simulink model "PMSM_FOC_INVERTER_COMPARISON"  (R2023b)
settings: Solver=VariableStepAuto  StartTime=0.0  StopTime=1  RelTol=1e-3
InitFcn:
  | Ld = 1.7e-3;
  | Lq = 3.2e-3;
  | Rs = 0.02;
  | Lambda_m = 0.2205;
  | J = 0.0027;
  | P = 4;
  | B = 0.001;
  | Vdc = 500;
libraries: slpidlib x9, spsControlledVoltageSourceLib x3, spsGroundLib x3, spsVoltageMeasurementLib x3, spsDCVoltageSourceLib x1, spsPermanentMagnetSynchronousMachineLib x1, spsUniversalBridgeLib x1, sps_lib x1, spsTriangleGeneratorLib x1
(part 1 of 2)
settings Model: Creator=Nabil  LastModifiedBy=Nabil

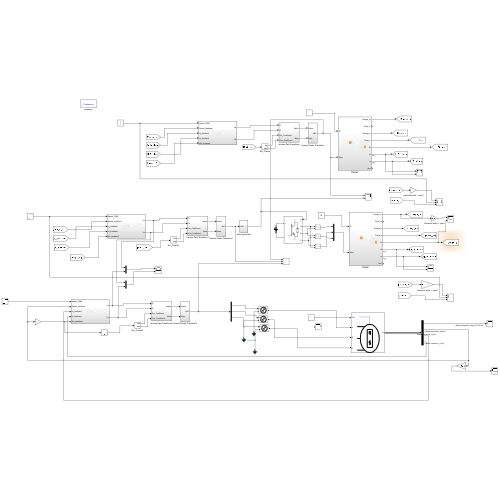
[thumbnail: Simulink's stored preview of the top-level diagram]
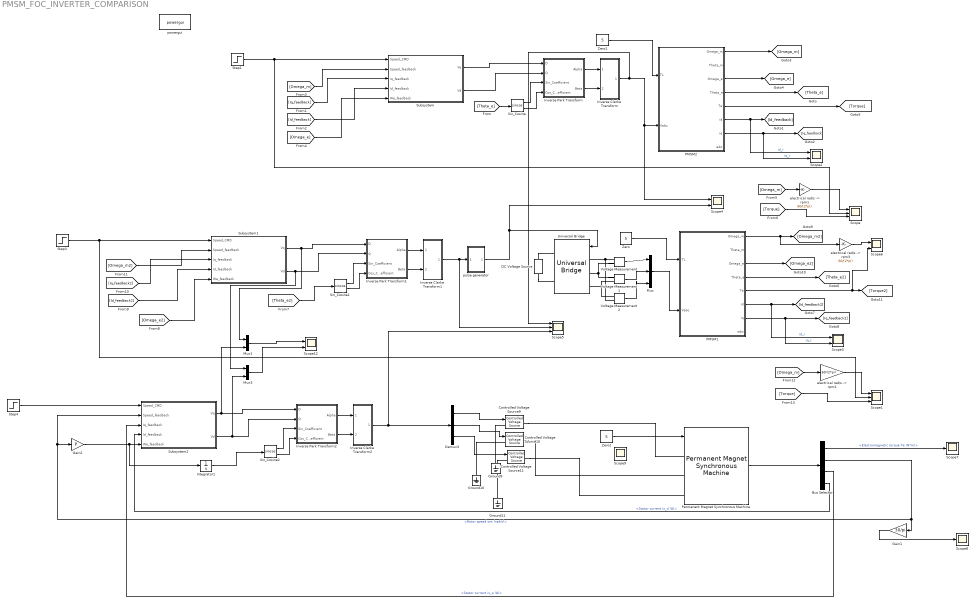
== system PMSM_FOC_INVERTER_COMPARISON ==
  Bus Selector : BusSelector  OutputSignals=Electromagnetic torque Te (N*m),Rotor speed wm (rad/s),Stator current is_q (A),Stator current is_d (A)
  Controlled Voltage Source10 : spsControlledVoltageSourceLib/Controlled Voltage Source  Initialize=on  Source_Type=AC  Amplitude=0  Phase=0  Frequency=0  Measurements=None
  Controlled Voltage Source11 : spsControlledVoltageSourceLib/Controlled Voltage Source  Initialize=on  Source_Type=AC  Amplitude=0  Phase=0  Frequency=0  Measurements=None
  Controlled Voltage Source9 : spsControlledVoltageSourceLib/Controlled Voltage Source  Initialize=on  Source_Type=AC  Amplitude=0  Phase=0  Frequency=0  Measurements=None
  DC Voltage Source : spsDCVoltageSourceLib/DC Voltage Source  Amplitude=Vdc  Measurements=None
  Demux3 : Demux  Outputs=3
  Gain1 : Gain  Gain=30/pi
  Gain2 : Gain  Gain=P
  Ground10 : spsGroundLib/Ground  LConnTagsString=a
  Ground11 : spsGroundLib/Ground  LConnTagsString=a
  Ground9 : spsGroundLib/Ground  LConnTagsString=a
  Integrator1 : Integrator
  Inverse Clarke Transform : Subsystem
  Inverse Clarke Transform1 : Subsystem
  Inverse Clarke Transform2 : Subsystem
  Inverse Park Transform : Subsystem
  Inverse Park Transform1 : Subsystem
  Inverse Park Transform2 : Subsystem
  Mux : Mux  Inputs=3
  Mux1 : Mux  Inputs=2
  Mux3 : Mux  Inputs=2
  PMSM1 : Subsystem
  PMSM2 : Subsystem
  Permanent Magnet Synchronous Machine : spsPermanentMagnetSynchronousMachineLib/Permanent Magnet Synchronous Machine  NbPhases=3  FluxDistribution=Sinusoidal  RotorType=Round  MechanicalLoad=Torque Tm  PresetModel=No  ShowDetailedParameters=on  MeasurementBus=off  Resistance=0.0485  Inductance=8.5e-3  dqInductances=[8.5e-3,8.5e-3]  La=0.000395  MachineConstant=Flux linkage established by magnets (V.s)  Flux=0.1194  VoltageCst=86.6271  TorqueCst=0.7164  Flat=120  Mechanical=[0.0027 0.0004924 4 0]  PolePairs=4  InitialConditions=[0,0, 0,0]  InitialConditions5ph=[0 0 0 0 0 0]  RefAngle=90 degrees behind phase A axis (modified Park)  IterativeDiscreteModel=Trapezoidal non iterative  TsBlock=-1  TsPowergui=0
  Scope : Scope  NumInputPorts=3
  Scope1 : Scope  NumInputPorts=3
  Scope{2..4,6,12} (5 alike) : Scope  NumInputPorts=2
  Scope5 : Scope  NumInputPorts=3
  Scope7 : Scope
  Scope8 : Scope
  Scope9 : Scope
  Sin_Cosine : Trigonometry  Operator=sincos
  Sin_Cosine1 : Trigonometry  Operator=sincos
  Sin_Cosine2 : Trigonometry  Operator=sincos
  Step1 : Step  Time=0.7  Before=500  After=1000  SampleTime=0
  Step3 : Step  Time=0.7  Before=500  After=1000  SampleTime=0
  Step4 : Step  Time=0.7  Before=500  After=1000  SampleTime=0
  Subsystem : Subsystem
  Subsystem1 : Subsystem
  Subsystem2 : Subsystem
  Universal Bridge : spsUniversalBridgeLib/Universal Bridge  Arms=3  SnubberResistance=1e5  SnubberCapacitance=inf  Device=IGBT / Diodes  Ron=1e-3  Lon=0  ForwardVoltages="[  0  0  ]"  ForwardVoltage=0  GTOparameters=[ 10e-6 , 20e-6 ]  IGBTparameters=[ 1e-6 , 2e-6 ]  Measurements=None  Measurements_2=None  converterType=Rectifier
  Voltage Measurement : spsVoltageMeasurementLib/Voltage Measurement  PhasorSimulation=off  OutputType=Complex  PSBequivalent=0
  Voltage Measurement1 : spsVoltageMeasurementLib/Voltage Measurement  PhasorSimulation=off  OutputType=Complex  PSBequivalent=0
  Voltage Measurement2 : spsVoltageMeasurementLib/Voltage Measurement  PhasorSimulation=off  OutputType=Complex  PSBequivalent=0
  Zero : Constant  Value=5  OutDataTypeStr=Inherit: Inherit via back propagation
  Zero1 : Constant  Value=5  OutDataTypeStr=Inherit: Inherit via back propagation
  Zero2 : Constant  Value=5  OutDataTypeStr=Inherit: Inherit via back propagation
  "electrical rad/s -> rpm1" : Gain  Gain=60/(2*pi)
  "electrical rad/s -> rpm2" : Gain  Gain=60/(2*pi)
  "electrical rad/s -> rpm3" : Gain  Gain=60/(2*pi)
  powergui : sps_lib/powergui  Priority=1  SimulationMode=Continuous  SampleTime=50e-6  frequency=60  Iterations=50  frequencyindice=0  Pbase=100e6  ErrMax=1e-4  UnitsV=kV  UnitsW=MW  buscounter=0  FunctionMessages=off  echomessages=off  EnableUseOfTLC=off  CurrentSourceSwitches=off  DisableSnubberDevices=off  DisableRonSwitches=off  DisableVfSwitches=off  DisplayEquations=off  AutomaticDiscreteSolvers=off  SolverType=Tustin/Backward Euler (TBE)  Interpol=off  ExternalGateDelay=off  methode=off  Ts=100  x0status=blocks  SPID=on  SwTol=0  HookPort=off  NonlinearTolerance=1e-4  nMaxIteration=100  ContinueOnMaxIteration=off  RestoreLinks=warning  ResistiveCurrentMeasurement=off  Frange=[0:2:500]  Ylog=off  Xlog=on  ShowGrid=off  save=off  variable=ZData  structure=0  ZoomFFT=off  StartTime=0.0  cycles=1  DisplayStyle=1  fundamental=60  FreqAxis=off  MaxFrequency=1000  frequencyindicesteady=1  RmsSteady=1  display=off
  pulse generator : Subsystem
  wires:
  [Theta_e] -> Sin_Cosine/1
  Sin_Cosine/2 -> Inverse Park Transform/4(Cos_Coefficient)
  Sin_Cosine/1 -> Inverse Park Transform/3(Sin_Coefficient)
  Inverse Park Transform/2(Beta) -> Inverse Clarke Transform/2(Beta)
  Inverse Park Transform/1(Alpha) -> Inverse Clarke Transform/1(Alpha)
  PMSM2/4(Theta_e) -> [Theta_e]
  Subsystem/1(Vq) -> Inverse Park Transform/1(D)
  Subsystem/2(Vd) -> Inverse Park Transform/2(Q)
  Step1/1 -> Scope/2, Subsystem/1(Speed_CMD)
  PMSM2/7(iq) -> Scope2/2, [Iq_feedback]  "iq_r"
  PMSM2/6(id) -> Scope2/1, [Id_feedback]  "id_r"
  [Iq_feedback] -> Subsystem/3(Iq_feedback)
  [Id_feedback] -> Subsystem/4(Id_feedback)
  PMSM2/1(Omega_m) -> [Omega_m]
  [Omega_m] -> Subsystem/2(Speed_feedback)
  PMSM2/3(Omega_e) -> [Omega_e]
  [Omega_e] -> Subsystem/5(We_feedback)
  PMSM2/5(Te) -> [Torque]
  [Torque] -> Scope/3
  Inverse Clarke Transform/1(ABC) -> Scope5/1, Scope4/1, PMSM2/2(Vabc)
  [Omega_m] -> "electrical rad/s -> rpm1"/1
  "electrical rad/s -> rpm1"/1 -> Scope/1
  "electrical rad/s -> rpm2"/1 -> Scope1/1
  [Omega_m] -> "electrical rad/s -> rpm2"/1
  [Torque] -> Scope1/3
  PMSM1/5(Te) -> Scope6/2, [Torque2]
  [Omega_e2] -> Subsystem1/5(We_feedback)
  PMSM1/3(Omega_e) -> [Omega_e2]
  [Omega_m2] -> Subsystem1/2(Speed_feedback)
  PMSM1/1(Omega_m) -> "electrical rad/s -> rpm3"/1, [Omega_m2]
  [Id_feedback2] -> Subsystem1/4(Id_feedback)
  [Iq_feedback2] -> Subsystem1/3(Iq_feedback)
  PMSM1/6(id) -> [Id_feedback2], Scope3/1  "id_r"
  PMSM1/7(iq) -> [Iq_feedback2], Scope3/2  "iq_r"
  Step3/1 -> Scope1/2, Subsystem1/1(Speed_CMD)
  Subsystem1/2(Vd) -> Mux3/1, Inverse Park Transform1/2(Q)
  Subsystem1/1(Vq) -> Mux1/1, Inverse Park Transform1/1(D)
  PMSM1/4(Theta_e) -> [Theta_e2]
  Inverse Park Transform1/1(Alpha) -> Inverse Clarke Transform1/1(Alpha)
  Inverse Park Transform1/2(Beta) -> Inverse Clarke Transform1/2(Beta)
  Sin_Cosine1/1 -> Inverse Park Transform1/3(Sin_Coefficient)
  Sin_Cosine1/2 -> Inverse Park Transform1/4(Cos_Coefficient)
  [Theta_e2] -> Sin_Cosine1/1
  Voltage Measurement/1 -> Mux/1
  Voltage Measurement1/1 -> Mux/2
  Voltage Measurement2/1 -> Mux/3
  Mux/1 -> PMSM1/2(Vabc)
  Inverse Clarke Transform1/1(ABC) -> Scope5/2, pulse generator/1(ABC)
  pulse generator/1(Out1) -> Universal Bridge/1, Scope4/2
  Zero/1 -> PMSM1/1(TL)
  Zero1/1 -> PMSM2/1(TL)
  "electrical rad/s -> rpm3"/1 -> Scope6/1
  Inverse Clarke Transform2/1(ABC) -> Scope5/3, Demux3/1
  Sin_Cosine2/2 -> Inverse Park Transform2/4(Cos_Coefficient)
  Sin_Cosine2/1 -> Inverse Park Transform2/3(Sin_Coefficient)
  Inverse Park Transform2/2(Beta) -> Inverse Clarke Transform2/2(Beta)
  Inverse Park Transform2/1(Alpha) -> Inverse Clarke Transform2/1(Alpha)
  Subsystem2/1(Vq) -> Mux1/2, Inverse Park Transform2/1(D)
  Subsystem2/2(Vd) -> Mux3/2, Inverse Park Transform2/2(Q)
  Zero2/1 -> Permanent Magnet Synchronous Machine/1
  Permanent Magnet Synchronous Machine/1 -> Bus Selector/1
  Bus Selector/1 -> Scope7/1  "<Electromagnetic torque Te (N*m)>"
  Bus Selector/2 -> Gain1/1, Subsystem2/2(Speed_feedback), Gain2/1  "<Rotor speed wm (rad/s)>"
  Bus Selector/3 -> Subsystem2/3(Iq_feedback)  "<Stator current is_q (A)>"
  Bus Selector/4 -> Subsystem2/4(Id_feedback)  "<Stator current is_d (A)>"
  Gain1/1 -> Scope8/1
  Gain2/1 -> Integrator1/1, Subsystem2/5(We_feedback)
  Integrator1/1 -> Sin_Cosine2/1
  Demux3/1 -> Controlled Voltage Source9/1
  Demux3/2 -> Controlled Voltage Source10/1
  Demux3/3 -> Controlled Voltage Source11/1
  Mux1/1 -> Scope12/1
  Mux3/1 -> Scope12/2
  Step4/1 -> Subsystem2/1(Speed_CMD)
  connections:
  DC Voltage Source/RConn1 -- Universal Bridge/RConn1
  DC Voltage Source/LConn1 -- Universal Bridge/RConn2
  Voltage Measurement/LConn1 -- Universal Bridge/LConn1 -- Voltage Measurement2/LConn2
  Voltage Measurement/LConn2 -- Voltage Measurement1/LConn1 -- Universal Bridge/LConn2
  Voltage Measurement1/LConn2 -- Voltage Measurement2/LConn1 -- Universal Bridge/LConn3
  Ground9/LConn1 -- Controlled Voltage Source9/LConn1
  Ground10/LConn1 -- Controlled Voltage Source10/LConn1
  Ground11/LConn1 -- Controlled Voltage Source11/LConn1
  Controlled Voltage Source9/RConn1 -- Permanent Magnet Synchronous Machine/LConn1
  Controlled Voltage Source10/RConn1 -- Permanent Magnet Synchronous Machine/LConn2
  Controlled Voltage Source11/RConn1 -- Permanent Magnet Synchronous Machine/LConn3

== system PMSM_FOC_INVERTER_COMPARISON/Inverse Clarke Transform ==
  note: Inverse Clarke Transform
  note: Converts direct axis (alpha) component and the quadrature axis (beta) component to balanced three-phase quantities
      | The alpha and beta components are dependent on time and speed.
  Alpha : Inport
  Beta : Inport  Port=2
  Add : Sum  Inputs=-+  OutDataTypeStr=Inherit: Same as first input
  Add1 : Sum  Inputs=--  OutDataTypeStr=Inherit: Same as first input
  Gain : Gain  Gain=1/2
  Gain1 : Gain  Gain=sqrt(3)/2
  Mux : Mux  Inputs=3
  ABC : Outport  VectorParamsAs1DForOutWhenUnconnected=off
  wires:
  Beta/1 -> Gain1/1
  Mux/1 -> ABC/1
  Alpha/1 -> Mux/1, Gain/1
  Add1/1 -> Mux/3
  Gain1/1 -> Add1/2, Add/2
  Gain/1 -> Add1/1, Add/1
  Add/1 -> Mux/2

== system PMSM_FOC_INVERTER_COMPARISON/Inverse Clarke Transform1 ==
  note: Converts direct axis (alpha) component and the quadrature axis (beta) component to balanced three-phase quantities
      | The alpha and beta components are dependent on time and speed.
  note: Inverse Clarke Transform
  Alpha : Inport
  Beta : Inport  Port=2
  Add : Sum  Inputs=-+  OutDataTypeStr=Inherit: Same as first input
  Add1 : Sum  Inputs=--  OutDataTypeStr=Inherit: Same as first input
  Gain : Gain  Gain=1/2
  Gain1 : Gain  Gain=sqrt(3)/2
  Mux : Mux  Inputs=3
  ABC : Outport  VectorParamsAs1DForOutWhenUnconnected=off
  wires:
  Add/1 -> Mux/2
  Gain/1 -> Add/1, Add1/1
  Gain1/1 -> Add/2, Add1/2
  Add1/1 -> Mux/3
  Alpha/1 -> Gain/1, Mux/1
  Mux/1 -> ABC/1
  Beta/1 -> Gain1/1

== system PMSM_FOC_INVERTER_COMPARISON/Inverse Clarke Transform2 ==
  note: Inverse Clarke Transform
  note: Converts direct axis (alpha) component and the quadrature axis (beta) component to balanced three-phase quantities
      | The alpha and beta components are dependent on time and speed.
  Alpha : Inport
  Beta : Inport  Port=2
  Add : Sum  Inputs=-+  OutDataTypeStr=Inherit: Same as first input
  Add1 : Sum  Inputs=--  OutDataTypeStr=Inherit: Same as first input
  Gain : Gain  Gain=1/2
  Gain1 : Gain  Gain=sqrt(3)/2
  Mux : Mux  Inputs=3
  ABC : Outport  VectorParamsAs1DForOutWhenUnconnected=off
  wires:
  Beta/1 -> Gain1/1
  Mux/1 -> ABC/1
  Alpha/1 -> Mux/1, Gain/1
  Add1/1 -> Mux/3
  Gain1/1 -> Add1/2, Add/2
  Gain/1 -> Add1/1, Add/1
  Add/1 -> Mux/2

== system PMSM_FOC_INVERTER_COMPARISON/Inverse Park Transform ==
  note: Converts orthogonal rotating reference frame (dq) to two-phase orthogonal stationary reference frame (alpha, beta)
  note: Inverse Park Transform
  D : Inport
  Q : Inport  Port=2
  Sin_Coefficient : Inport  Port=3
  Cos_Coefficient : Inport  Port=4
  Add1 : Sum  Inputs=+-  OutDataTypeStr=Inherit: Same as first input
  Add2 : Sum  OutDataTypeStr=Inherit: Same as first input
  Cos_Coefficient_1 : InportShadow  Port=4
  Product{1..4} (4 alike) : Product  RndMeth=Simplest
  Sin_Coefficient_1 : InportShadow  Port=3
  Alpha : Outport  VectorParamsAs1DForOutWhenUnconnected=off
  Beta : Outport  Port=2  VectorParamsAs1DForOutWhenUnconnected=off
  wires:
  Sin_Coefficient_1/1 -> Product3/2
  Product2/1 -> Add1/2
  Cos_Coefficient_1/1 -> Product4/2
  Add2/1 -> Beta/1
  Product3/1 -> Add2/1
  Add1/1 -> Alpha/1
  Product1/1 -> Add1/1
  Product4/1 -> Add2/2
  Sin_Coefficient/1 -> Product2/2
  D/1 -> Product3/1, Product1/1
  Q/1 -> Product2/1, Product4/1
  Cos_Coefficient/1 -> Product1/2

== system PMSM_FOC_INVERTER_COMPARISON/Inverse Park Transform1 ==
  note: Inverse Park Transform
  note: Converts orthogonal rotating reference frame (dq) to two-phase orthogonal stationary reference frame (alpha, beta)
  D : Inport
  Q : Inport  Port=2
  Sin_Coefficient : Inport  Port=3
  Cos_Coefficient : Inport  Port=4
  Add1 : Sum  Inputs=+-  OutDataTypeStr=Inherit: Same as first input
  Add2 : Sum  OutDataTypeStr=Inherit: Same as first input
  Cos_Coefficient_1 : InportShadow  Port=4
  Product{1..4} (4 alike) : Product  RndMeth=Simplest
  Sin_Coefficient_1 : InportShadow  Port=3
  Alpha : Outport  VectorParamsAs1DForOutWhenUnconnected=off
  Beta : Outport  Port=2  VectorParamsAs1DForOutWhenUnconnected=off
  wires:
  Cos_Coefficient/1 -> Product1/2
  Q/1 -> Product4/1, Product2/1
  D/1 -> Product1/1, Product3/1
  Sin_Coefficient/1 -> Product2/2
  Product4/1 -> Add2/2
  Product1/1 -> Add1/1
  Add1/1 -> Alpha/1
  Product3/1 -> Add2/1
  Add2/1 -> Beta/1
  Cos_Coefficient_1/1 -> Product4/2
  Product2/1 -> Add1/2
  Sin_Coefficient_1/1 -> Product3/2

== system PMSM_FOC_INVERTER_COMPARISON/Inverse Park Transform2 ==
  note: Converts orthogonal rotating reference frame (dq) to two-phase orthogonal stationary reference frame (alpha, beta)
  note: Inverse Park Transform
  D : Inport
  Q : Inport  Port=2
  Sin_Coefficient : Inport  Port=3
  Cos_Coefficient : Inport  Port=4
  Add1 : Sum  Inputs=+-  OutDataTypeStr=Inherit: Same as first input
  Add2 : Sum  OutDataTypeStr=Inherit: Same as first input
  Cos_Coefficient_1 : InportShadow  Port=4
  Product{1..4} (4 alike) : Product  RndMeth=Simplest
  Sin_Coefficient_1 : InportShadow  Port=3
  Alpha : Outport  VectorParamsAs1DForOutWhenUnconnected=off
  Beta : Outport  Port=2  VectorParamsAs1DForOutWhenUnconnected=off
  wires:
  Sin_Coefficient_1/1 -> Product3/2
  Product2/1 -> Add1/2
  Cos_Coefficient_1/1 -> Product4/2
  Add2/1 -> Beta/1
  Product3/1 -> Add2/1
  Add1/1 -> Alpha/1
  Product1/1 -> Add1/1
  Product4/1 -> Add2/2
  Sin_Coefficient/1 -> Product2/2
  D/1 -> Product3/1, Product1/1
  Q/1 -> Product2/1, Product4/1
  Cos_Coefficient/1 -> Product1/2

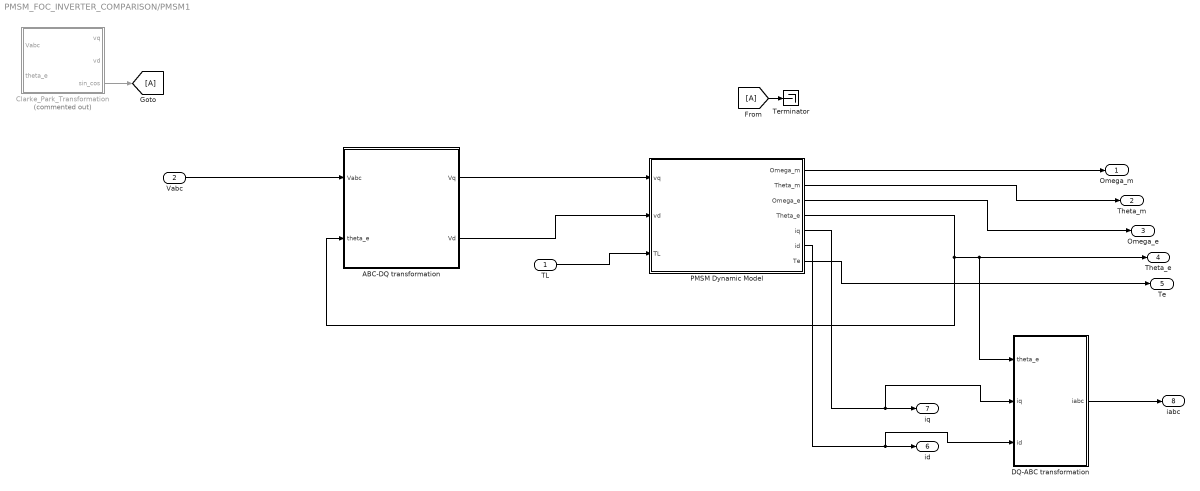
== system PMSM_FOC_INVERTER_COMPARISON/PMSM1 ==
  TL : Inport
  Vabc : Inport  Port=2
  ABC-DQ transformation : Subsystem
  Clarke_Park_Transformation : Subsystem  Commented=on
  DQ-ABC transformation : Subsystem
  From : From
  Goto : Goto
  PMSM Dynamic Model : Subsystem
  Terminator : Terminator
  Omega_m : Outport
  Theta_m : Outport  Port=2
  Omega_e : Outport  Port=3
  Theta_e : Outport  Port=4
  Te : Outport  Port=5
  id : Outport  Port=6
  iq : Outport  Port=7
  iabc : Outport  Port=8
  wires:
  DQ-ABC transformation/1(iabc) -> iabc/1
  ABC-DQ transformation/2(Vd) -> PMSM Dynamic Model/2(vd)
  ABC-DQ transformation/1(Vq) -> PMSM Dynamic Model/1(vq)
  Vabc/1 -> ABC-DQ transformation/1(Vabc)
  PMSM Dynamic Model/3(Omega_e) -> Omega_e/1
  PMSM Dynamic Model/1(Omega_m) -> Omega_m/1
  TL/1 -> PMSM Dynamic Model/3(TL)
  PMSM Dynamic Model/4(Theta_e) -> Theta_e/1, DQ-ABC transformation/1(theta_e), ABC-DQ transformation/2(theta_e)
  Clarke_Park_Transformation/3(sin_cos) -> Goto/1
  PMSM Dynamic Model/5(iq) -> iq/1, DQ-ABC transformation/2(iq)
  PMSM Dynamic Model/6(id) -> id/1, DQ-ABC transformation/3(id)
  PMSM Dynamic Model/7(Te) -> Te/1
  PMSM Dynamic Model/2(Theta_m) -> Theta_m/1
  From/1 -> Terminator/1

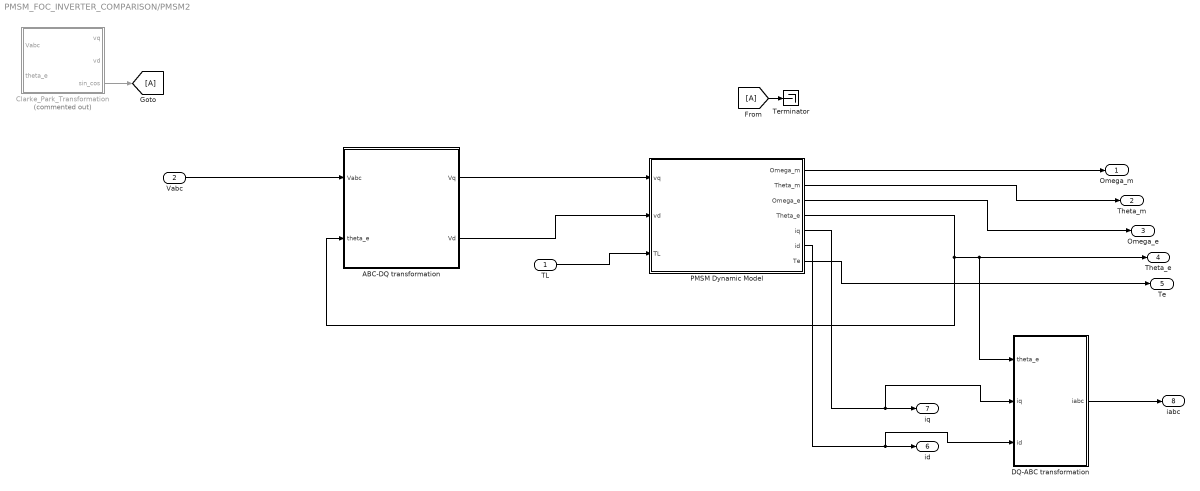
== system PMSM_FOC_INVERTER_COMPARISON/PMSM2 ==
  TL : Inport
  Vabc : Inport  Port=2
  ABC-DQ transformation : Subsystem
  Clarke_Park_Transformation : Subsystem  Commented=on
  DQ-ABC transformation : Subsystem
  From : From
  Goto : Goto
  PMSM Dynamic Model : Subsystem
  Terminator : Terminator
  Omega_m : Outport
  Theta_m : Outport  Port=2
  Omega_e : Outport  Port=3
  Theta_e : Outport  Port=4
  Te : Outport  Port=5
  id : Outport  Port=6
  iq : Outport  Port=7
  iabc : Outport  Port=8
  wires:
  From/1 -> Terminator/1
  PMSM Dynamic Model/2(Theta_m) -> Theta_m/1
  PMSM Dynamic Model/7(Te) -> Te/1
  PMSM Dynamic Model/6(id) -> DQ-ABC transformation/3(id), id/1
  PMSM Dynamic Model/5(iq) -> DQ-ABC transformation/2(iq), iq/1
  Clarke_Park_Transformation/3(sin_cos) -> Goto/1
  PMSM Dynamic Model/4(Theta_e) -> ABC-DQ transformation/2(theta_e), DQ-ABC transformation/1(theta_e), Theta_e/1
  TL/1 -> PMSM Dynamic Model/3(TL)
  PMSM Dynamic Model/1(Omega_m) -> Omega_m/1
  PMSM Dynamic Model/3(Omega_e) -> Omega_e/1
  Vabc/1 -> ABC-DQ transformation/1(Vabc)
  ABC-DQ transformation/1(Vq) -> PMSM Dynamic Model/1(vq)
  ABC-DQ transformation/2(Vd) -> PMSM Dynamic Model/2(vd)
  DQ-ABC transformation/1(iabc) -> iabc/1

== system PMSM_FOC_INVERTER_COMPARISON/Subsystem ==
  Speed_CMD : Inport
  Speed_feedback : Inport  Port=2
  Iq_feedback : Inport  Port=3
  Id_feedback : Inport  Port=4
  We_feedback : Inport  Port=5
  Current Controller : Subsystem
  Subsystem : Subsystem
  "electrical rad/s -> rpm1" : Gain  Gain=60/(2*pi)
  Vq : Outport
  Vd : Outport  Port=2
  wires:
  Speed_CMD/1 -> Subsystem/1(Speed_CMD)
  Subsystem/1(Iq_ref) -> Current Controller/1(iq_reference)
  Subsystem/2(Id_ref) -> Current Controller/2(id_reference)
  We_feedback/1 -> Current Controller/5(spd_we)
  Current Controller/1(vd_reference) -> Vq/1
  Current Controller/2(vq_reference) -> Vd/1
  Iq_feedback/1 -> Current Controller/4(iq_feedback)
  Id_feedback/1 -> Current Controller/3(id_feedback)
  Speed_feedback/1 -> "electrical rad/s -> rpm1"/1
  "electrical rad/s -> rpm1"/1 -> Subsystem/2(Speed_feedback)

== system PMSM_FOC_INVERTER_COMPARISON/Subsystem1 ==
  Speed_CMD : Inport
  Speed_feedback : Inport  Port=2
  Iq_feedback : Inport  Port=3
  Id_feedback : Inport  Port=4
  We_feedback : Inport  Port=5
  Current Controller : Subsystem
  Subsystem : Subsystem
  "electrical rad/s -> rpm1" : Gain  Gain=60/(2*pi)
  Vq : Outport
  Vd : Outport  Port=2
  wires:
  "electrical rad/s -> rpm1"/1 -> Subsystem/2(Speed_feedback)
  Speed_feedback/1 -> "electrical rad/s -> rpm1"/1
  Id_feedback/1 -> Current Controller/3(id_feedback)
  Iq_feedback/1 -> Current Controller/4(iq_feedback)
  Current Controller/2(vq_reference) -> Vd/1
  Current Controller/1(vd_reference) -> Vq/1
  We_feedback/1 -> Current Controller/5(spd_we)
  Subsystem/2(Id_ref) -> Current Controller/2(id_reference)
  Subsystem/1(Iq_ref) -> Current Controller/1(iq_reference)
  Speed_CMD/1 -> Subsystem/1(Speed_CMD)

== system PMSM_FOC_INVERTER_COMPARISON/Subsystem2 ==
  Speed_CMD : Inport
  Speed_feedback : Inport  Port=2
  Iq_feedback : Inport  Port=3
  Id_feedback : Inport  Port=4
  We_feedback : Inport  Port=5
  Current Controller : Subsystem
  Subsystem : Subsystem
  "electrical rad/s -> rpm1" : Gain  Gain=60/(2*pi)
  Vq : Outport
  Vd : Outport  Port=2
  wires:
  Speed_CMD/1 -> Subsystem/1(Speed_CMD)
  Subsystem/1(Iq_ref) -> Current Controller/1(iq_reference)
  Subsystem/2(Id_ref) -> Current Controller/2(id_reference)
  We_feedback/1 -> Current Controller/5(spd_we)
  Current Controller/1(vd_reference) -> Vq/1
  Current Controller/2(vq_reference) -> Vd/1
  Iq_feedback/1 -> Current Controller/4(iq_feedback)
  Id_feedback/1 -> Current Controller/3(id_feedback)
  Speed_feedback/1 -> "electrical rad/s -> rpm1"/1
  "electrical rad/s -> rpm1"/1 -> Subsystem/2(Speed_feedback)

== system PMSM_FOC_INVERTER_COMPARISON/pulse generator ==
  ABC : Inport
  Demux : Demux  Outputs=3
  Gain : Gain  Gain=1/Vdc
  Gain1 : Gain  Gain=1/Vdc
  Gain2 : Gain  Gain=1/Vdc
  Mux : Mux  Inputs=6
  NOT : Logic  Operator=NOT  IconShape=distinctive  AllPortsSameDT=off  OutDataTypeStr=boolean
  NOT1 : Logic  Operator=NOT  IconShape=distinctive  AllPortsSameDT=off  OutDataTypeStr=boolean
  NOT2 : Logic  Operator=NOT  IconShape=distinctive  AllPortsSameDT=off  OutDataTypeStr=boolean
  Relational Operator : RelationalOperator  OutDataTypeStr=boolean  RndMeth=Simplest  InputSameDT=off
  Relational Operator1 : RelationalOperator  OutDataTypeStr=boolean  RndMeth=Simplest  InputSameDT=off
  Relational Operator2 : RelationalOperator  OutDataTypeStr=boolean  RndMeth=Simplest  InputSameDT=off
  Triangle Generator : spsTriangleGeneratorLib/Triangle Generator  Freq=1e4  Phase=0  Ts=0
  Out1 : Outport
  wires:
  Gain/1 -> Relational Operator/1
  Demux/2 -> Gain1/1
  Demux/3 -> Gain2/1
  Gain2/1 -> Relational Operator2/1
  Gain1/1 -> Relational Operator1/1
  Triangle Generator/1 -> Relational Operator/2, Relational Operator1/2, Relational Operator2/2
  Relational Operator/1 -> Mux/1, NOT/1
  NOT/1 -> Mux/2
  Relational Operator1/1 -> Mux/3, NOT1/1
  NOT1/1 -> Mux/4
  Relational Operator2/1 -> Mux/5, NOT2/1
  NOT2/1 -> Mux/6
  Mux/1 -> Out1/1
  ABC/1 -> Demux/1
  Demux/1 -> Gain/1

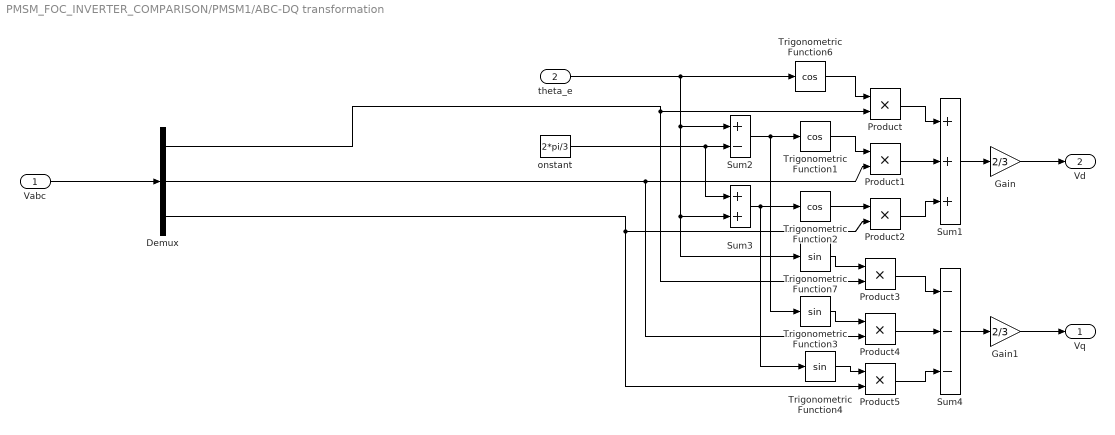
== system PMSM_FOC_INVERTER_COMPARISON/PMSM1/ABC-DQ transformation ==
  Vabc : Inport
  theta_e : Inport  Port=2
  Demux : Demux  Outputs=3
  Gain : Gain  Gain=2/3
  Gain1 : Gain  Gain=2/3
  Product{,1..5} (6 alike) : Product  RndMeth=Zero
  Sum1 : Sum  Inputs=+++  InputSameDT=on  SaturateOnIntegerOverflow=on  OutDataTypeStr=Inherit: Same as first input
  Sum2 : Sum  Inputs=+-  InputSameDT=on  SaturateOnIntegerOverflow=on  OutDataTypeStr=Inherit: Same as first input
  Sum3 : Sum  InputSameDT=on  SaturateOnIntegerOverflow=on  OutDataTypeStr=Inherit: Same as first input
  Sum4 : Sum  Inputs=---  InputSameDT=on  SaturateOnIntegerOverflow=on  OutDataTypeStr=Inherit: Same as first input
  Trigonometric Function1 : Trigonometry  Operator=cos
  Trigonometric Function2 : Trigonometry  Operator=cos
  Trigonometric Function3 : Trigonometry
  Trigonometric Function4 : Trigonometry
  Trigonometric Function6 : Trigonometry  Operator=cos
  Trigonometric Function7 : Trigonometry
  onstant : Constant  Value=2*pi/3
  Vq : Outport
  Vd : Outport  Port=2
  wires:
  Vabc/1 -> Demux/1
  Product/1 -> Sum1/1
  Trigonometric Function6/1 -> Product/1
  Trigonometric Function4/1 -> Product5/1
  Product4/1 -> Sum4/2
  Sum1/1 -> Gain/1
  Trigonometric Function1/1 -> Product1/1
  Product2/1 -> Sum1/3
  Trigonometric Function2/1 -> Product2/1
  Trigonometric Function7/1 -> Product3/1
  theta_e/1 -> Sum3/2, Trigonometric Function7/1, Sum2/1, Trigonometric Function6/1
  Product1/1 -> Sum1/2
  Sum3/1 -> Trigonometric Function4/1, Trigonometric Function2/1
  Sum2/1 -> Trigonometric Function3/1, Trigonometric Function1/1
  Trigonometric Function3/1 -> Product4/1
  Sum4/1 -> Gain1/1
  onstant/1 -> Sum3/1, Sum2/2
  Gain1/1 -> Vq/1
  Demux/3 -> Product5/2, Product2/2
  Product3/1 -> Sum4/1
  Demux/2 -> Product4/2, Product1/2
  Demux/1 -> Product3/2, Product/2
  Product5/1 -> Sum4/3
  Gain/1 -> Vd/1

== system PMSM_FOC_INVERTER_COMPARISON/PMSM1/Clarke_Park_Transformation ==
  Vabc : Inport
  theta_e : Inport  Port=2
  Clarke Transformation : Subsystem
  Constant4 : Constant  Value=0
  Mux : Mux  Inputs=2
  Park Transformation : Subsystem
  Subsystem : Subsystem
  Terminator : Terminator
  vq : Outport
  vd : Outport  Port=2
  sin_cos : Outport  Port=3
  wires:
  theta_e/1 -> Subsystem/1(theta_e)
  Subsystem/2(sin) -> Mux/2, Park Transformation/4(Sin theta_e)
  Park Transformation/1(qs_r) -> vq/1
  Clarke Transformation/2(vd_s) -> Park Transformation/2(ds_s)
  Clarke Transformation/1(vq_s) -> Park Transformation/1(qs_s)
  Subsystem/1(cos) -> Mux/1, Park Transformation/3(cos theta_e)
  Clarke Transformation/3(vo_s) -> Terminator/1
  Park Transformation/2(ds_r) -> vd/1
  Constant4/1 -> Clarke Transformation/2(theta_degree)
  Mux/1 -> sin_cos/1
  Vabc/1 -> Clarke Transformation/1(abc)

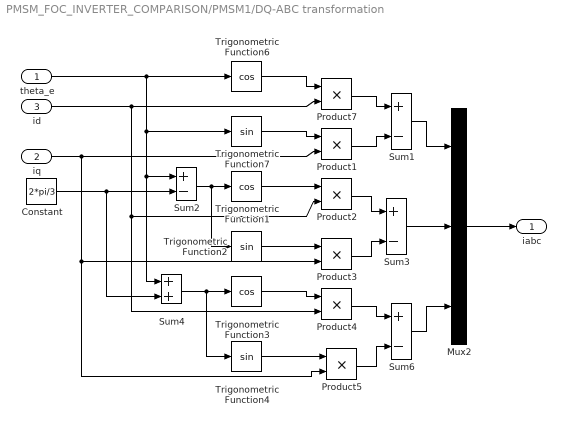
== system PMSM_FOC_INVERTER_COMPARISON/PMSM1/DQ-ABC transformation ==
  theta_e : Inport
  iq : Inport  Port=2
  id : Inport  Port=3
  Constant : Constant  Value=2*pi/3
  Mux2 : Mux  Inputs=3
  Product{1..5,7} (6 alike) : Product  InputSameDT=on  RndMeth=Zero  SaturateOnIntegerOverflow=on  OutDataTypeStr=Inherit: Same as first input
  Sum{1..3,6} (4 alike) : Sum  Inputs=+-  InputSameDT=on  SaturateOnIntegerOverflow=on  OutDataTypeStr=Inherit: Same as first input
  Sum4 : Sum  InputSameDT=on  SaturateOnIntegerOverflow=on  OutDataTypeStr=Inherit: Same as first input
  Trigonometric Function1 : Trigonometry  Operator=cos
  Trigonometric Function2 : Trigonometry
  Trigonometric Function3 : Trigonometry  Operator=cos
  Trigonometric Function4 : Trigonometry
  Trigonometric Function6 : Trigonometry  Operator=cos
  Trigonometric Function7 : Trigonometry
  iabc : Outport
  wires:
  Product7/1 -> Sum1/1
  Product1/1 -> Sum1/2
  Product4/1 -> Sum6/1
  Sum3/1 -> Mux2/2
  Sum6/1 -> Mux2/3
  Trigonometric Function1/1 -> Product2/1
  id/1 -> Product4/2, Product2/2, Product7/2
  theta_e/1 -> Sum4/1, Sum2/1, Trigonometric Function7/1, Trigonometric Function6/1
  Trigonometric Function6/1 -> Product7/1
  Trigonometric Function2/1 -> Product3/1
  Sum4/1 -> Trigonometric Function4/1, Trigonometric Function3/1
  Trigonometric Function3/1 -> Product4/1
  Product3/1 -> Sum3/2
  Product5/1 -> Sum6/2
  Sum1/1 -> Mux2/1
  Mux2/1 -> iabc/1
  Trigonometric Function7/1 -> Product1/1
  Constant/1 -> Sum4/2, Sum2/2
  Trigonometric Function4/1 -> Product5/1
  iq/1 -> Product5/2, Product3/2, Product1/2
  Sum2/1 -> Trigonometric Function2/1, Trigonometric Function1/1
  Product2/1 -> Sum3/1

== system PMSM_FOC_INVERTER_COMPARISON/PMSM1/PMSM Dynamic Model ==
  vq : Inport
  vd : Inport  Port=2
  TL : Inport  Port=3
  Electromagnetic Torque : Subsystem
  Subsystem : Subsystem
  iqd_calculations : Subsystem
  Omega_m : Outport
  Theta_m : Outport  Port=2
  Omega_e : Outport  Port=3
  Theta_e : Outport  Port=4
  iq : Outport  Port=5
  id : Outport  Port=6
  Te : Outport  Port=7
  wires:
  vd/1 -> iqd_calculations/3(vd)
  vq/1 -> iqd_calculations/1(vq)
  Subsystem/2(Theta_m) -> Theta_m/1
  Subsystem/1(Omega_m) -> Omega_m/1
  iqd_calculations/2(id) -> Electromagnetic Torque/2(id), id/1
  iqd_calculations/1(iq) -> Electromagnetic Torque/1(iq), iq/1
  Subsystem/4(Theta_e) -> Theta_e/1
  TL/1 -> Subsystem/2(TL)
  Electromagnetic Torque/1(Te) -> Subsystem/1(Te), Te/1
  Subsystem/3(Omega_e) -> iqd_calculations/2(Omega_e), Omega_e/1

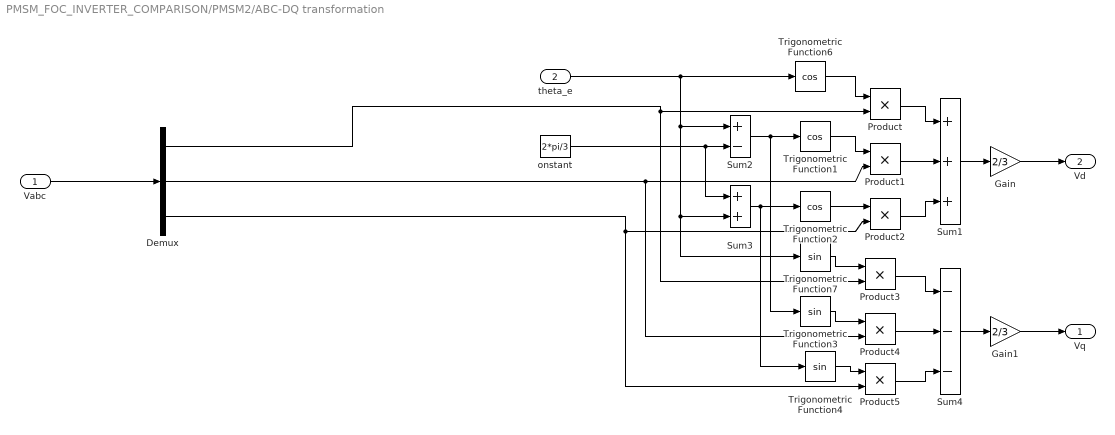
== system PMSM_FOC_INVERTER_COMPARISON/PMSM2/ABC-DQ transformation ==
  Vabc : Inport
  theta_e : Inport  Port=2
  Demux : Demux  Outputs=3
  Gain : Gain  Gain=2/3
  Gain1 : Gain  Gain=2/3
  Product{,1..5} (6 alike) : Product  RndMeth=Zero
  Sum1 : Sum  Inputs=+++  InputSameDT=on  SaturateOnIntegerOverflow=on  OutDataTypeStr=Inherit: Same as first input
  Sum2 : Sum  Inputs=+-  InputSameDT=on  SaturateOnIntegerOverflow=on  OutDataTypeStr=Inherit: Same as first input
  Sum3 : Sum  InputSameDT=on  SaturateOnIntegerOverflow=on  OutDataTypeStr=Inherit: Same as first input
  Sum4 : Sum  Inputs=---  InputSameDT=on  SaturateOnIntegerOverflow=on  OutDataTypeStr=Inherit: Same as first input
  Trigonometric Function1 : Trigonometry  Operator=cos
  Trigonometric Function2 : Trigonometry  Operator=cos
  Trigonometric Function3 : Trigonometry
  Trigonometric Function4 : Trigonometry
  Trigonometric Function6 : Trigonometry  Operator=cos
  Trigonometric Function7 : Trigonometry
  onstant : Constant  Value=2*pi/3
  Vq : Outport
  Vd : Outport  Port=2
  wires:
  Gain/1 -> Vd/1
  Product5/1 -> Sum4/3
  Demux/1 -> Product/2, Product3/2
  Demux/2 -> Product1/2, Product4/2
  Product3/1 -> Sum4/1
  Demux/3 -> Product2/2, Product5/2
  Gain1/1 -> Vq/1
  onstant/1 -> Sum2/2, Sum3/1
  Sum4/1 -> Gain1/1
  Trigonometric Function3/1 -> Product4/1
  Sum2/1 -> Trigonometric Function1/1, Trigonometric Function3/1
  Sum3/1 -> Trigonometric Function2/1, Trigonometric Function4/1
  Product1/1 -> Sum1/2
  theta_e/1 -> Trigonometric Function6/1, Sum2/1, Trigonometric Function7/1, Sum3/2
  Trigonometric Function7/1 -> Product3/1
  Trigonometric Function2/1 -> Product2/1
  Product2/1 -> Sum1/3
  Trigonometric Function1/1 -> Product1/1
  Sum1/1 -> Gain/1
  Product4/1 -> Sum4/2
  Trigonometric Function4/1 -> Product5/1
  Trigonometric Function6/1 -> Product/1
  Product/1 -> Sum1/1
  Vabc/1 -> Demux/1

== system PMSM_FOC_INVERTER_COMPARISON/PMSM2/Clarke_Park_Transformation ==
  Vabc : Inport
  theta_e : Inport  Port=2
  Clarke Transformation : Subsystem
  Constant4 : Constant  Value=0
  Mux : Mux  Inputs=2
  Park Transformation : Subsystem
  Subsystem : Subsystem
  Terminator : Terminator
  vq : Outport
  vd : Outport  Port=2
  sin_cos : Outport  Port=3
  wires:
  Vabc/1 -> Clarke Transformation/1(abc)
  Mux/1 -> sin_cos/1
  Constant4/1 -> Clarke Transformation/2(theta_degree)
  Park Transformation/2(ds_r) -> vd/1
  Clarke Transformation/3(vo_s) -> Terminator/1
  Subsystem/1(cos) -> Park Transformation/3(cos theta_e), Mux/1
  Clarke Transformation/1(vq_s) -> Park Transformation/1(qs_s)
  Clarke Transformation/2(vd_s) -> Park Transformation/2(ds_s)
  Park Transformation/1(qs_r) -> vq/1
  Subsystem/2(sin) -> Park Transformation/4(Sin theta_e), Mux/2
  theta_e/1 -> Subsystem/1(theta_e)

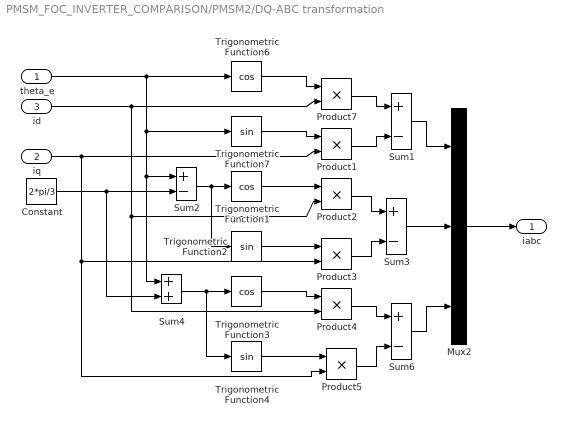
== system PMSM_FOC_INVERTER_COMPARISON/PMSM2/DQ-ABC transformation ==
  theta_e : Inport
  iq : Inport  Port=2
  id : Inport  Port=3
  Constant : Constant  Value=2*pi/3
  Mux2 : Mux  Inputs=3
  Product{1..5,7} (6 alike) : Product  InputSameDT=on  RndMeth=Zero  SaturateOnIntegerOverflow=on  OutDataTypeStr=Inherit: Same as first input
  Sum{1..3,6} (4 alike) : Sum  Inputs=+-  InputSameDT=on  SaturateOnIntegerOverflow=on  OutDataTypeStr=Inherit: Same as first input
  Sum4 : Sum  InputSameDT=on  SaturateOnIntegerOverflow=on  OutDataTypeStr=Inherit: Same as first input
  Trigonometric Function1 : Trigonometry  Operator=cos
  Trigonometric Function2 : Trigonometry
  Trigonometric Function3 : Trigonometry  Operator=cos
  Trigonometric Function4 : Trigonometry
  Trigonometric Function6 : Trigonometry  Operator=cos
  Trigonometric Function7 : Trigonometry
  iabc : Outport
  wires:
  Product2/1 -> Sum3/1
  Sum2/1 -> Trigonometric Function1/1, Trigonometric Function2/1
  iq/1 -> Product1/2, Product3/2, Product5/2
  Trigonometric Function4/1 -> Product5/1
  Constant/1 -> Sum2/2, Sum4/2
  Trigonometric Function7/1 -> Product1/1
  Mux2/1 -> iabc/1
  Sum1/1 -> Mux2/1
  Product5/1 -> Sum6/2
  Product3/1 -> Sum3/2
  Trigonometric Function3/1 -> Product4/1
  Sum4/1 -> Trigonometric Function3/1, Trigonometric Function4/1
  Trigonometric Function2/1 -> Product3/1
  Trigonometric Function6/1 -> Product7/1
  theta_e/1 -> Trigonometric Function6/1, Trigonometric Function7/1, Sum2/1, Sum4/1
  id/1 -> Product7/2, Product2/2, Product4/2
  Trigonometric Function1/1 -> Product2/1
  Sum6/1 -> Mux2/3
  Sum3/1 -> Mux2/2
  Product4/1 -> Sum6/1
  Product1/1 -> Sum1/2
  Product7/1 -> Sum1/1

== system PMSM_FOC_INVERTER_COMPARISON/PMSM2/PMSM Dynamic Model ==
  vq : Inport
  vd : Inport  Port=2
  TL : Inport  Port=3
  Electromagnetic Torque : Subsystem
  Subsystem : Subsystem
  iqd_calculations : Subsystem
  Omega_m : Outport
  Theta_m : Outport  Port=2
  Omega_e : Outport  Port=3
  Theta_e : Outport  Port=4
  iq : Outport  Port=5
  id : Outport  Port=6
  Te : Outport  Port=7
  wires:
  Subsystem/3(Omega_e) -> Omega_e/1, iqd_calculations/2(Omega_e)
  Electromagnetic Torque/1(Te) -> Te/1, Subsystem/1(Te)
  TL/1 -> Subsystem/2(TL)
  Subsystem/4(Theta_e) -> Theta_e/1
  iqd_calculations/1(iq) -> iq/1, Electromagnetic Torque/1(iq)
  iqd_calculations/2(id) -> id/1, Electromagnetic Torque/2(id)
  Subsystem/1(Omega_m) -> Omega_m/1
  Subsystem/2(Theta_m) -> Theta_m/1
  vq/1 -> iqd_calculations/1(vq)
  vd/1 -> iqd_calculations/3(vd)

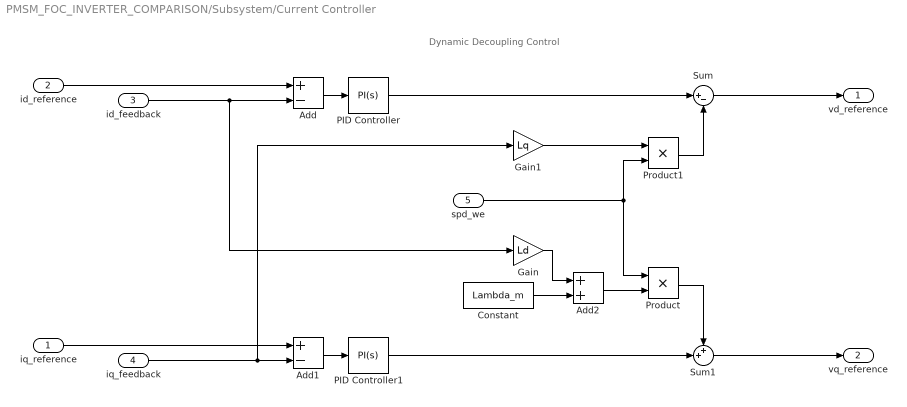
== system PMSM_FOC_INVERTER_COMPARISON/Subsystem/Current Controller ==
  note: Dynamic Decoupling Control
  iq_reference : Inport  SampleTime=1e-4
  id_reference : Inport  Port=2  SampleTime=1e-4
  id_feedback : Inport  Port=3  SampleTime=1e-4
  iq_feedback : Inport  Port=4  SampleTime=1e-4
  spd_we : Inport  Port=5  SampleTime=1e-4
  Add : Sum  Inputs=+-
  Add1 : Sum  Inputs=+-
  Add2 : Sum
  Constant : Constant  Value=Lambda_m  SampleTime=1e-4
  Gain : Gain  Gain=Ld
  Gain1 : Gain  Gain=Lq
  PID Controller : slpidlib/PID Controller  Controller=PI  Form=Parallel  TimeDomain=Continuous-time  UseExternalTs=off  SampleTime=-1  IntegratorMethod=Forward Euler  FilterMethod=Forward Euler  ControllerParametersSource=internal  P=7.74  I=26.84  UseKiTs=off  D=0  N=100  UseFilter=on  TunerSelectOption=Transfer Function Based (PID Tuner App)  InitialConditionSource=internal  InitialConditionForIntegrator=0  InitialConditionForFilter=0  DifferentiatorICPrevScaledInput=0  ExternalReset=none  TrackingMode=off  Kt=1  LimitOutput=off  SatLimitsSource=internal  UpperSaturationLimit=inf  LowerSaturationLimit=-inf  LinearizeAsGain=on  AntiWindupMode=none  Kb=1  LimitIntegrator=off  UpperIntegratorSaturationLimit=inf  LowerIntegratorSaturationLimit=-inf  POutMin=[]  POutMax=[]  IOutMin=[]  IOutMax=[]  DOutMin=[]  DOutMax=[]  NOutMin=[]  NOutMax=[]  SumOutMin=[]  SumOutMax=[]  SaturationOutMin=[]  SaturationOutMax=[]  PParamMin=[]  PParamMax=[]  IParamMin=[]  IParamMax=[]  DParamMin=[]  DParamMax=[]  NParamMin=[]  NParamMax=[]  KbParamMin=[]  KbParamMax=[]  KtParamMin=[]  KtParamMax=[]  KbOutMin=[]  KbOutMax=[]  KtOutMin=[]  KtOutMax=[]  IntegratorOutMin=[]  IntegratorOutMax=[]  FilterOutMin=[]  FilterOutMax=[]  SumI1OutMin=[]  SumI1OutMax=[]  SumI2OutMin=[]  SumI2OutMax=[]  SumI3OutMin=[]  SumI3OutMax=[]  SumI4OutMin=[]  SumI4OutMax=[]  SumDOutMin=[]  SumDOutMax=[]  DifferentiatorOutMin=[]  DifferentiatorOutMax=[]  FilterDiffOutCoefMin=[]  FilterDiffOutCoefMax=[]  ReciprocalOutMin=[]  ReciprocalOutMax=[]  SumDenOutMin=[]  SumDenOutMax=[]  SumNumOutMin=[]  SumNumOutMax=[]  DivideOutMin=[]  DivideOutMax=[]  UdiffTsProdOutMin=[]  UdiffTsProdOutMax=[]  NTsProdOutMin=[]  NTsProdOutMax=[]  UintegralTsProdOutMin=[]  UintegralTsProdOutMax=[]  UngainTsProdOutMin=[]  UngainTsProdOutMax=[]  ClampingZeroOutDataTypeStr=Inherit: Inherit via back propagation  ClampingZeroOutMin=[]  ClampingZeroOutMax=[]  FilterDenConstantOutDataTypeStr=Inherit: Inherit via back propagation  FilterDenConstantOutMin=[]  FilterDenConstantOutMax=[]  PCopyOutDataTypeStr=Inherit: Inherit via back propagation  PCopyOutMin=[]  PCopyOutMax=[]  NCopyOutDataTypeStr=Inherit: Inherit via back propagation  NCopyOutMin=[]  NCopyOutMax=[]  IntegratorContinuousStateAttributes=''  IntegratorStateMustResolveToSignalObject=off  IntegratorRTWStateStorageClass=Auto  FilterContinuousStateAttributes=''  FilterStateMustResolveToSignalObject=off  FilterRTWStateStorageClass=Auto  ParallelPVariant=InternalParameters  IdealPVariant=Disabled  IVariant=InternalParameters  DVariant=Disabled  IntegratorVariant=Continuous  SatVariant=Disabled  AWVariant=Passthrough  PCopyVariant=Disabled  TRVariant=Disabled  FdbkBlocksVariant=Forward  IdealPFdbkVariant=Disabled  SatFdbkVariant=Disabled  DerivativeFilterVariant=Disabled  NVariant=Disabled  NCopyVariant=Disabled_SignalSpec  FilterICVariant=Disabled  IntegratorICVariant=InternalICs  ExternalResetVariant=Disabled  TRSumVariant=Passthrough  SumFdbkVariant=Disabled  SumVariant=Sum_PI  TsampFilterVariant=InternalTs  TsampNgainVariant=Passthrough  TsampIntegralVariant=Disabled_SignalSpec  ExternalSaturationOutDataTypeStr=Inherit: Same as second input
  PID Controller1 : slpidlib/PID Controller  Controller=PI  Form=Parallel  TimeDomain=Continuous-time  UseExternalTs=off  SampleTime=-1  IntegratorMethod=Forward Euler  FilterMethod=Forward Euler  ControllerParametersSource=internal  P=7.74  I=26.84  UseKiTs=off  D=0  N=100  UseFilter=on  TunerSelectOption=Transfer Function Based (PID Tuner App)  InitialConditionSource=internal  InitialConditionForIntegrator=0  InitialConditionForFilter=0  DifferentiatorICPrevScaledInput=0  ExternalReset=none  TrackingMode=off  Kt=1  LimitOutput=off  SatLimitsSource=internal  UpperSaturationLimit=inf  LowerSaturationLimit=-inf  LinearizeAsGain=on  AntiWindupMode=none  Kb=1  LimitIntegrator=off  UpperIntegratorSaturationLimit=inf  LowerIntegratorSaturationLimit=-inf  POutMin=[]  POutMax=[]  IOutMin=[]  IOutMax=[]  DOutMin=[]  DOutMax=[]  NOutMin=[]  NOutMax=[]  SumOutMin=[]  SumOutMax=[]  SaturationOutMin=[]  SaturationOutMax=[]  PParamMin=[]  PParamMax=[]  IParamMin=[]  IParamMax=[]  DParamMin=[]  DParamMax=[]  NParamMin=[]  NParamMax=[]  KbParamMin=[]  KbParamMax=[]  KtParamMin=[]  KtParamMax=[]  KbOutMin=[]  KbOutMax=[]  KtOutMin=[]  KtOutMax=[]  IntegratorOutMin=[]  IntegratorOutMax=[]  FilterOutMin=[]  FilterOutMax=[]  SumI1OutMin=[]  SumI1OutMax=[]  SumI2OutMin=[]  SumI2OutMax=[]  SumI3OutMin=[]  SumI3OutMax=[]  SumI4OutMin=[]  SumI4OutMax=[]  SumDOutMin=[]  SumDOutMax=[]  DifferentiatorOutMin=[]  DifferentiatorOutMax=[]  FilterDiffOutCoefMin=[]  FilterDiffOutCoefMax=[]  ReciprocalOutMin=[]  ReciprocalOutMax=[]  SumDenOutMin=[]  SumDenOutMax=[]  SumNumOutMin=[]  SumNumOutMax=[]  DivideOutMin=[]  DivideOutMax=[]  UdiffTsProdOutMin=[]  UdiffTsProdOutMax=[]  NTsProdOutMin=[]  NTsProdOutMax=[]  UintegralTsProdOutMin=[]  UintegralTsProdOutMax=[]  UngainTsProdOutMin=[]  UngainTsProdOutMax=[]  ClampingZeroOutDataTypeStr=Inherit: Inherit via back propagation  ClampingZeroOutMin=[]  ClampingZeroOutMax=[]  FilterDenConstantOutDataTypeStr=Inherit: Inherit via back propagation  FilterDenConstantOutMin=[]  FilterDenConstantOutMax=[]  PCopyOutDataTypeStr=Inherit: Inherit via back propagation  PCopyOutMin=[]  PCopyOutMax=[]  NCopyOutDataTypeStr=Inherit: Inherit via back propagation  NCopyOutMin=[]  NCopyOutMax=[]  IntegratorContinuousStateAttributes=''  IntegratorStateMustResolveToSignalObject=off  IntegratorRTWStateStorageClass=Auto  FilterContinuousStateAttributes=''  FilterStateMustResolveToSignalObject=off  FilterRTWStateStorageClass=Auto  ParallelPVariant=InternalParameters  IdealPVariant=Disabled  IVariant=InternalParameters  DVariant=Disabled  IntegratorVariant=Continuous  SatVariant=Disabled  AWVariant=Passthrough  PCopyVariant=Disabled  TRVariant=Disabled  FdbkBlocksVariant=Forward  IdealPFdbkVariant=Disabled  SatFdbkVariant=Disabled  DerivativeFilterVariant=Disabled  NVariant=Disabled  NCopyVariant=Disabled_SignalSpec  FilterICVariant=Disabled  IntegratorICVariant=InternalICs  ExternalResetVariant=Disabled  TRSumVariant=Passthrough  SumFdbkVariant=Disabled  SumVariant=Sum_PI  TsampFilterVariant=InternalTs  TsampNgainVariant=Passthrough  TsampIntegralVariant=Disabled_SignalSpec  ExternalSaturationOutDataTypeStr=Inherit: Same as second input
  Product : Product
  Product1 : Product
  Sum : Sum  Inputs=|+-
  Sum1 : Sum  Inputs=++|
  vd_reference : Outport  SampleTime=1e-4  VectorParamsAs1DForOutWhenUnconnected=off
  vq_reference : Outport  Port=2  SampleTime=1e-4  VectorParamsAs1DForOutWhenUnconnected=off
  wires:
  Sum/1 -> vd_reference/1
  PID Controller/1 -> Sum/1
  id_feedback/1 -> Gain/1, Add/2
  Add/1 -> PID Controller/1
  iq_feedback/1 -> Gain1/1, Add1/2
  id_reference/1 -> Add/1
  Add1/1 -> PID Controller1/1
  iq_reference/1 -> Add1/1
  Sum1/1 -> vq_reference/1
  PID Controller1/1 -> Sum1/2
  Gain/1 -> Add2/1
  Constant/1 -> Add2/2
  Add2/1 -> Product/2
  spd_we/1 -> Product1/2, Product/1
  Gain1/1 -> Product1/1
  Product1/1 -> Sum/2
  Product/1 -> Sum1/1

== system PMSM_FOC_INVERTER_COMPARISON/Subsystem/Subsystem ==
  Speed_CMD : Inport
  Speed_feedback : Inport  Port=2
  Gain : Gain  Gain=2/(3*P*Lambda_m)
  Id_CMD : Constant  Value=0
  PID Controller1 : slpidlib/PID Controller  Controller=PI  Form=Parallel  TimeDomain=Continuous-time  UseExternalTs=off  SampleTime=-1  IntegratorMethod=Forward Euler  FilterMethod=Forward Euler  ControllerParametersSource=internal  P=0.232686365732661  I=3.18596000308125  UseKiTs=off  D=0  N=100  UseFilter=on  TunerSelectOption=Transfer Function Based (PID Tuner App)  InitialConditionSource=internal  InitialConditionForIntegrator=0  InitialConditionForFilter=0  DifferentiatorICPrevScaledInput=0  ExternalReset=none  TrackingMode=off  Kt=1  LimitOutput=off  SatLimitsSource=internal  UpperSaturationLimit=inf  LowerSaturationLimit=-inf  LinearizeAsGain=on  AntiWindupMode=none  Kb=1  LimitIntegrator=off  UpperIntegratorSaturationLimit=inf  LowerIntegratorSaturationLimit=-inf  POutMin=[]  POutMax=[]  IOutMin=[]  IOutMax=[]  DOutMin=[]  DOutMax=[]  NOutMin=[]  NOutMax=[]  SumOutMin=[]  SumOutMax=[]  SaturationOutMin=[]  SaturationOutMax=[]  PParamMin=[]  PParamMax=[]  IParamMin=[]  IParamMax=[]  DParamMin=[]  DParamMax=[]  NParamMin=[]  NParamMax=[]  KbParamMin=[]  KbParamMax=[]  KtParamMin=[]  KtParamMax=[]  KbOutMin=[]  KbOutMax=[]  KtOutMin=[]  KtOutMax=[]  IntegratorOutMin=[]  IntegratorOutMax=[]  FilterOutMin=[]  FilterOutMax=[]  SumI1OutMin=[]  SumI1OutMax=[]  SumI2OutMin=[]  SumI2OutMax=[]  SumI3OutMin=[]  SumI3OutMax=[]  SumI4OutMin=[]  SumI4OutMax=[]  SumDOutMin=[]  SumDOutMax=[]  DifferentiatorOutMin=[]  DifferentiatorOutMax=[]  FilterDiffOutCoefMin=[]  FilterDiffOutCoefMax=[]  ReciprocalOutMin=[]  ReciprocalOutMax=[]  SumDenOutMin=[]  SumDenOutMax=[]  SumNumOutMin=[]  SumNumOutMax=[]  DivideOutMin=[]  DivideOutMax=[]  UdiffTsProdOutMin=[]  UdiffTsProdOutMax=[]  NTsProdOutMin=[]  NTsProdOutMax=[]  UintegralTsProdOutMin=[]  UintegralTsProdOutMax=[]  UngainTsProdOutMin=[]  UngainTsProdOutMax=[]  ClampingZeroOutDataTypeStr=Inherit: Inherit via back propagation  ClampingZeroOutMin=[]  ClampingZeroOutMax=[]  FilterDenConstantOutDataTypeStr=Inherit: Inherit via back propagation  FilterDenConstantOutMin=[]  FilterDenConstantOutMax=[]  PCopyOutDataTypeStr=Inherit: Inherit via back propagation  PCopyOutMin=[]  PCopyOutMax=[]  NCopyOutDataTypeStr=Inherit: Inherit via back propagation  NCopyOutMin=[]  NCopyOutMax=[]  IntegratorContinuousStateAttributes=''  IntegratorStateMustResolveToSignalObject=off  IntegratorRTWStateStorageClass=Auto  FilterContinuousStateAttributes=''  FilterStateMustResolveToSignalObject=off  FilterRTWStateStorageClass=Auto  ParallelPVariant=InternalParameters  IdealPVariant=Disabled  IVariant=InternalParameters  DVariant=Disabled  IntegratorVariant=Continuous  SatVariant=Disabled  AWVariant=Passthrough  PCopyVariant=Disabled  TRVariant=Disabled  FdbkBlocksVariant=Forward  IdealPFdbkVariant=Disabled  SatFdbkVariant=Disabled  DerivativeFilterVariant=Disabled  NVariant=Disabled  NCopyVariant=Disabled_SignalSpec  FilterICVariant=Disabled  IntegratorICVariant=InternalICs  ExternalResetVariant=Disabled  TRSumVariant=Passthrough  SumFdbkVariant=Disabled  SumVariant=Sum_PI  TsampFilterVariant=InternalTs  TsampNgainVariant=Passthrough  TsampIntegralVariant=Disabled_SignalSpec  ExternalSaturationOutDataTypeStr=Inherit: Same as second input
  Sum : Sum  Inputs=|+-
  Iq_ref : Outport
  Id_ref : Outport  Port=2
  wires:
  Speed_feedback/1 -> Sum/2
  Sum/1 -> PID Controller1/1
  Speed_CMD/1 -> Sum/1
  Id_CMD/1 -> Id_ref/1
  PID Controller1/1 -> Gain/1
  Gain/1 -> Iq_ref/1
